simulink model "Flexible_Beam_LP"  (R2014a)
settings: Solver=ode23t  StartTime=0.0  StopTime=200  RelTol=1e-3  AbsTol=1e-6
PreLoadFcn:
  | Cantilever_Beam_MS2G_Parameters
PostLoadFcn:
  | warning off Simulink:Engine:UsingDefaultMaxStepSize
  | warning off Simulink:Engine:SaveWithParameterizedLinks_Warning
undefined symbols (not defined in the file): beam_length, beam_wall, beam_width, Damping, density, Extr_Data_Box, kbendingx, kbendingy, kelongz, ktwistz, num_elem, shearM, X, Y, youngsM, Z
libraries: sm_lib x307, nesl_utility x65
(part 1 of 9)
Description:
  | Copyright 2014 The MathWorks, Inc.
settings Model: Creator=smiller  LastModifiedBy=smiller
settings DebuggingCC: UnderspecifiedInitializationDetection=Classic  StateNameClashWarn=warning
settings ExplorerConfigSet: InternalSimMechanicsExplorerSettings="<ExplorerConfiguration><canonicalview>default</canonicalview><AnimationSetting><BasePlaybackSpeed>1.0</BasePlaybackSpeed><PlaybackSpeedFactor>1.0</PlaybackSpeedFactor></AnimationSetting><TilePanel><TileInfo><Tiles Columns=\"1\" Count=\"1\" Rows=\"1\"><Column Left=\"2\" Weight=\"1\"/><Column Left=\"626\"/><Row Top=\"2\" Weight=\"1\"/><Row Top=\"393\"/><Tile Height=\"1\" Width=\"1\" X=\"0\" Y=\"0\"/></Tiles></TileInfo><SceneInfo><SceneViewer><BGColor><R>0.60000002384185791</R><G>0.60000002384185791</G><B>0.60000002384185791</B></BGColor><Camera><Position><X>46.619711055341185</X><Y>-0.34983005837123721</Y><Z>0.38649668367083467</Z></Position><Center><X>15.061424751729401</X><Y>-0.47805428343950285</Y><Z>0.22325866927449958</Z></Center><Up><X>-0.0040752125209600008</X><Y>0.99998893056788307</Y><Z>0.0023518895830039648</Z></Up><Left>-1.9626362085342408</Left><Right>1.9626362085342408</Right><Bottom>-0.98671855330467229</Bottom><Top>0.98671855330467229</Top></Camera></SceneViewer></SceneInfo></TilePanel></ExplorerConfiguration>"

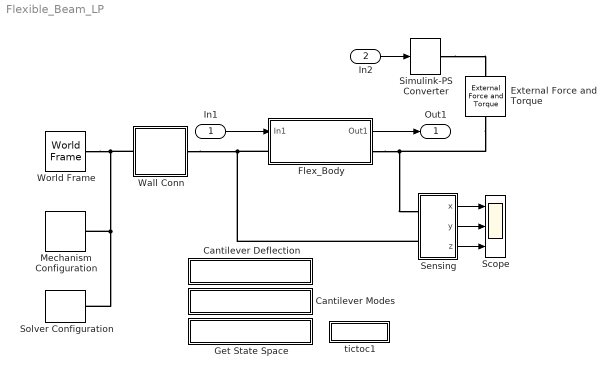
== system Flexible_Beam_LP ==
  In1 : Inport
  In2 : Inport  Port=2
  Cantilever Deflection : Subsystem
      settings: OpenFcn=|
      | mdl = bdroot;
      | 
      | load_system('FlexBeamElement_MS2G_Lib')
      | set_param('FlexBeamElement_MS2G_Lib', 'Lock', 'off');
      | set_param('FlexBeamElement_MS2G_Lib/Flex_Element','BlockChoice','Full')
      | 
      | open_system(mdl);
      | open_system([mdl, '/Scope']);
      | set_param([bdroot '/Wall Conn'],'OverrideUsingVariant','Fixed');
      | %set_param([mdl, '/Sensing/Transform Sensor'],'MeasurementFrame','World')
      | 
      | sim(mdl);
      | disp(['Static Deflection is ' num2str(TipDef.signals(2).values(end)) ' m'])
      mask Display: disp('Cantilever Deflection');
  Cantilever Modes : Subsystem
      settings: OpenFcn=Cantilever_Modes_Shapes_MS2G
      mask Display: disp('Cantilever Modes');
  External Force and Torque : sm_lib/Forces and Torques/External Force and Torque  ForceResolutionFrame=AttachedFrame  EnableForceX=off  EnableForceY=on  EnableForceZ=off  EnableForce=off  TorqueResolutionFrame=AttachedFrame  EnableTorqueX=off  EnableTorqueY=off  EnableTorqueZ=off  EnableTorque=off  BlockFunction=simmechanics.library.forces_torques.external_force_torque
  Flex_Body : Subsystem  mask(Flexible Body){rho=density, youngsM=youngsM, shearM=shearM, numelem=num_elem, beam_length=beam_length, beam_width=beam_width, beam_wall=beam_wall, b=Damping}
      mask prompts: rho "Material Density (kg/(m^3)"; youngsM "Modulus of Elasticity (N/m2)"; shearM "Shear Modulus (N/m2)"; numelem "Number of elements"; beam_length "Beam Length (m)"; beam_width "Beam Width & Height (m)"; beam_wall "Beam Wall Thickness(m)"; b "Damping Constant (Nm/rad.s)"
      mask help:
      | Models a flexible hollow square beam based on lumped parameter method.
      | Number of flexible elements, material properties as well as beam
      | dimension can be varied from mask parameters.
      mask init:
      | [kbendingx, kbendingy, ktwistz, kelongz, length] = Compute_GFE_Prop(rho, youngsM, shearM, numelem, beam_length, beam_width,beam_wall);
      | thisblock = gcb;
      | anno = ['No of Elem: ' num2str(numelem)];
      | set_param(thisblock, 'AttributesFormatString',anno);
      | set_param([thisblock '/Matrix Concatenate'],'NumInputs','numelem')
      | blkchoice = get_param('FlexBeamElement_MS2G_Lib/Flex_Element','BlockChoice');
      | if numelem <1
      |     error('Number of Flexible elements should be greater than 0')
      | end
      | prev_flex_bod = find_system(gcb,'LookUnderMasks','all','RegExp','on','Name','Flex_Elem_*');
      | if ~isempty(prev_flex_bod)
      |     delete_block(prev_flex_bod(1:end))
      | end
      | linehan = find_system(thisblock,'LookUnderMasks','all','FindAll','on','type','line');
      | if ~isempty(linehan)
      |     delete_line(linehan)
      | end
      | blk_or = [100 155 140 195];
      | set_param([thisblock '/B'],'Position',blk_or)
      | set_param([thisblock '/' sprintf('Transform\nBeamX')],'Position',blk_or+[80 0 80 0])
      | add_line(thisblock,['B/Rconn1'],[sprintf('Transform\nBeamX') '/Lconn1'],'autorouting','on');
      | add_block('FlexBeamElement_MS2G_Lib/Flex_Element',[thisblock '/Flex_Elem_' num2str(1)],'Position',blk_or+[80 0 80 0]*2)
      | add_line(thisblock,[sprintf('Transform\nBeamX') '/Rconn1'],['Flex_Elem_' num2str(1) '/Lconn1'],'autorouting','on');
      | add_line(thisblock,'In1/1',['Flex_Elem_' num2str(1) '/1'],'autorouting','on')
      | add_line(thisblock,['Flex_Elem_' num2str(1) '/1'],'Matrix Concatenate/1','autorouting','on')
      | set_param([thisblock '/Flex_Elem_' num2str(1)], 'LinkStatus', 'none')
      | set_param([thisblock '/Flex_Elem_' num2str(1) '/' blkchoice], 'LinkStatus', 'none')
      | set_param([thisblock '/Flex_Elem_' num2str(1) '/' blkchoice '/Selector'],'InputPortWidth','3*numelem')
      | set_param([thisblock '/Flex_Elem_' num2str(1) '/' blkchoice '/Selector'],'Indices','[1 2 3]')
      | if strcmp(blkchoice,'Full')
      |     state_order{1} = [thisblock '/Flex_Elem_' num2str(1) '/' blkchoice '/Bearing Joint'];
      | elseif strcmp(blkchoice,'Elong')
      |     state_order{1} = [thisblock '/Flex_Elem_' num2str(1) '/' blkchoice '/Prismatic Joint'];
      | else
      |     state_order{1} = [thisblock '/Flex_Elem_' num2str(1) '/' blkchoice '/Revolute Joint'];
      | end
      | for i = 2:1:numelem
      |     add_block('FlexBeamElement_MS2G_Lib/Flex_Element',[thisblock '/Flex_Elem_' num2str(i)],'Position',blk_or+(i+1)*[80 0 80 0])
      |     add_line(thisblock,['Flex_Elem_' num2str(i-1) '/Rconn1'],['Flex_Elem_' num2str(i) '/Lconn1'],'autorouting','on');
      |     add_line(thisblock,'In1/1',['Flex_Elem_' num2str(i) '/1'],'autorouting','on')
      |     add_line(thisblock,['Flex_Elem_' num2str(i) '/1'],['Matrix Concatenate/' num2str(i)],'autorouting','on')
      |     set_param([thisblock '/Flex_Elem_' num2str(i)], 'LinkStatus', 'none')
      |     set_param([thisblock '/Flex_Elem_' num2str(i) '/' blkchoice], 'LinkStatus', 'none')
      |     set_param([thisblock '/Flex_Elem_' num2str(i) '/' blkchoice '/Selector'],'InputPortWidth','3*numelem')
      |     set_param([thisblock '/Flex_Elem_' num2str(i) '/' blkchoice '/Selector'],'Indices',['[' num2str([3*i-2 3*i-1 3*i]) ']'])
      |     if strcmp(blkchoice,'Full')
      |         state_order{i} = [thisblock '/Flex_Elem_' num2str(i) '/' blkchoice '/Bearing Joint'];
      |     elseif strcmp(blkchoice,'Elong')
      |         state_order{i} = [thisblock '/Flex_Elem_' num2str(i) '/' blkchoice '/Prismatic Joint'];
      |     else
      |         state_order{i} = [thisblock '/Flex_Elem_' num2str(i) '/' blkchoice '/Revolute Joint'];
      |     end
      | end
      | set_param([thisblock '/F'],'Position',blk_or+ (numelem+2)*[80 0 80 0]);
      | add_line(thisblock,['Flex_Elem_' num2str(numelem) '/Rconn1'],['F/Rconn1'],'autorouting','on');
      | assignin('base','State_order',state_order)
      | add_line(thisblock,'Matrix Concatenate/1','Out1/1','autorouting','on')
      settings: AttributesFormatString=No of Elem: 30  CopyFcn=set_param(gcb, 'LinkStatus', 'none')
      mask Display:
      | image(imread('Flexible_Beam.png'));
      | port_label('input',1,'F_L');
      | port_label('output',1,'wz');
      | color red
      | port_label('LConn',1,'B');
      | port_label('RConn',1,'F');
  Get State Space : Subsystem
      settings: OpenFcn=Cantilever_Linearization_SS_Models
      mask Display: disp('Get State Space');
  Mechanism Configuration : sm_lib/Utilities/Mechanism Configuration  UniformGravity=Constant  GravityVector=gravity  GravityUnits=m/s^2  LinearizationDelta=0.001  BlockFunction=simmechanics.library.utilities.mechanism_configuration
  Scope : Scope  NumInputPorts=3
      settings: YMin=29.8~-1.5~-0.001  YMax=30.2~0~0.001  SaveName=TipDef
  Sensing : Subsystem
  Simulink-PS Converter : nesl_utility/Simulink-PS Converter  PhysicalDomain=network_engine_domain  SubClassName=ps_input  LeftPortType=input  RightPortType=output  PseudoPeriodic=off  Frequencies=[]  NoiseDistribution=none  NoiseParameters=[]  Unit=1  AffineConversion=off  InputFiltering=off  SimscapeFilterOrder=1  InputFilterTimeConstant=0.001  UdotUserProvided=1
  Solver Configuration : nesl_utility/Solver Configuration  PhysicalDomain=network_engine_domain  SubClassName=solver  LeftPortType=input  RightPortType=generic  Accelerate=off  Tones=[]  Harmonics=[]  SimulateNoise=off  Profile=off  UseLocalSampling=off  EnableSwitchedLinearOptims=on  FrequencyDomain=off  UseCCode=off  RelTol=0.001  AbsTol=1e-06  MinStep=1e-09  ToWorkspace=off  DoDC=off  ResidualTolerance=1e-09  UseLocalSolver=off  LocalSolverChoice=NE_BACKWARD_EULER_ADVANCER  LocalSolverSampleTime=0.001  DoFixedCost=off  MaxNonlinIter=3  MaxModeIter=2  LinearAlgebra=Sparse  DelaysMemoryBudget=1024  AutomaticFiltering=on  FilteringTimeConstant=0.001
  Wall Conn : Subsystem  Variant=on  OverrideUsingVariant=Fixed
      mask Display:
      | if strcmp(get_param(gcb,'ActiveVariant'),'Fixed')
      |     image(imread('Weld_Image.png'))
      | else
      |     image(imread('Rev_Image.png'))
      | end
      | color red
      | port_label('LConn',1,'B');
      | port_label('Rconn',1,'F');
  World Frame : sm_lib/Frames and Transforms/World Frame  BlockFunction=simmechanics.library.frames_transforms.world_frame
  tictoc1 : Subsystem
      settings: OpenFcn=open('Flexible_Beam_Demo_Script.html')
      mask Display: disp('Script')
  Out1 : Outport
  wires:
  In2/1 -> Simulink-PS Converter/1
  Sensing/1(x) -> Scope/1
  Sensing/2(y) -> Scope/2
  Sensing/3(z) -> Scope/3
  In1/1 -> Flex_Body/1(In1)
  Flex_Body/1(Out1) -> Out1/1
  connections:
  Simulink-PS Converter/RConn1 -- External Force and Torque/LConn1
  External Force and Torque/RConn1 -- Flex_Body/RConn1 -- Sensing/LConn1
  Solver Configuration/RConn1 -- Wall Conn/LConn1 -- World Frame/RConn1 -- Mechanism Configuration/RConn1
  Sensing/LConn2 -- Flex_Body/LConn1 -- Wall Conn/RConn1

== system Flexible_Beam_LP/Cantilever Deflection ==

== system Flexible_Beam_LP/Cantilever Modes ==

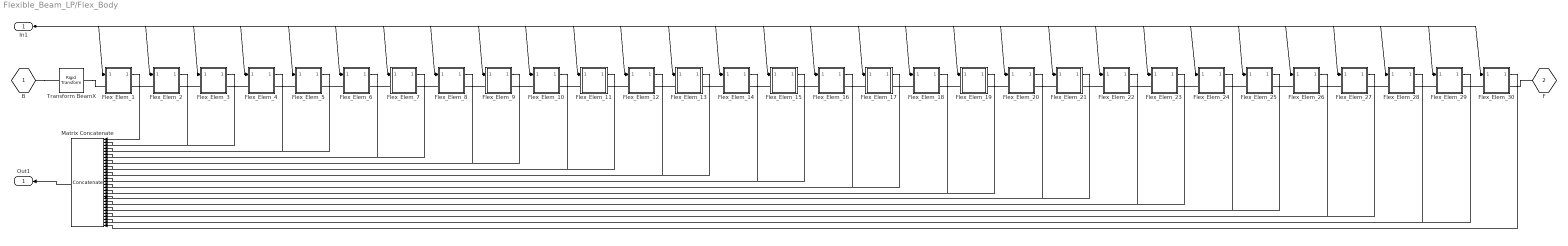
== system Flexible_Beam_LP/Flex_Body ==
  In1 : Inport
  Flex_Elem_1 : Subsystem  BlockChoice=Full
      settings: AttributesFormatString=%<BlockChoice>  TemplateBlock=FlexBeamElement_MS2G_Lib/Flex_Element  MemberBlocks=Bend,Elong,Full
  Flex_Elem_10 : Subsystem  BlockChoice=Full
      settings: AttributesFormatString=%<BlockChoice>  TemplateBlock=FlexBeamElement_MS2G_Lib/Flex_Element  MemberBlocks=Bend,Elong,Full
  Flex_Elem_11 : Subsystem  BlockChoice=Full
      settings: AttributesFormatString=%<BlockChoice>  TemplateBlock=FlexBeamElement_MS2G_Lib/Flex_Element  MemberBlocks=Bend,Elong,Full
  Flex_Elem_12 : Subsystem  BlockChoice=Full
      settings: AttributesFormatString=%<BlockChoice>  TemplateBlock=FlexBeamElement_MS2G_Lib/Flex_Element  MemberBlocks=Bend,Elong,Full
  Flex_Elem_13 : Subsystem  BlockChoice=Full
      settings: AttributesFormatString=%<BlockChoice>  TemplateBlock=FlexBeamElement_MS2G_Lib/Flex_Element  MemberBlocks=Bend,Elong,Full
  Flex_Elem_14 : Subsystem  BlockChoice=Full
      settings: AttributesFormatString=%<BlockChoice>  TemplateBlock=FlexBeamElement_MS2G_Lib/Flex_Element  MemberBlocks=Bend,Elong,Full
  Flex_Elem_15 : Subsystem  BlockChoice=Full
      settings: AttributesFormatString=%<BlockChoice>  TemplateBlock=FlexBeamElement_MS2G_Lib/Flex_Element  MemberBlocks=Bend,Elong,Full
  Flex_Elem_16 : Subsystem  BlockChoice=Full
      settings: AttributesFormatString=%<BlockChoice>  TemplateBlock=FlexBeamElement_MS2G_Lib/Flex_Element  MemberBlocks=Bend,Elong,Full
  Flex_Elem_17 : Subsystem  BlockChoice=Full
      settings: AttributesFormatString=%<BlockChoice>  TemplateBlock=FlexBeamElement_MS2G_Lib/Flex_Element  MemberBlocks=Bend,Elong,Full
  Flex_Elem_18 : Subsystem  BlockChoice=Full
      settings: AttributesFormatString=%<BlockChoice>  TemplateBlock=FlexBeamElement_MS2G_Lib/Flex_Element  MemberBlocks=Bend,Elong,Full
  Flex_Elem_19 : Subsystem  BlockChoice=Full
      settings: AttributesFormatString=%<BlockChoice>  TemplateBlock=FlexBeamElement_MS2G_Lib/Flex_Element  MemberBlocks=Bend,Elong,Full
  Flex_Elem_2 : Subsystem  BlockChoice=Full
      settings: AttributesFormatString=%<BlockChoice>  TemplateBlock=FlexBeamElement_MS2G_Lib/Flex_Element  MemberBlocks=Bend,Elong,Full
  Flex_Elem_20 : Subsystem  BlockChoice=Full
      settings: AttributesFormatString=%<BlockChoice>  TemplateBlock=FlexBeamElement_MS2G_Lib/Flex_Element  MemberBlocks=Bend,Elong,Full
  Flex_Elem_21 : Subsystem  BlockChoice=Full
      settings: AttributesFormatString=%<BlockChoice>  TemplateBlock=FlexBeamElement_MS2G_Lib/Flex_Element  MemberBlocks=Bend,Elong,Full
  Flex_Elem_22 : Subsystem  BlockChoice=Full
      settings: AttributesFormatString=%<BlockChoice>  TemplateBlock=FlexBeamElement_MS2G_Lib/Flex_Element  MemberBlocks=Bend,Elong,Full
  Flex_Elem_23 : Subsystem  BlockChoice=Full
      settings: AttributesFormatString=%<BlockChoice>  TemplateBlock=FlexBeamElement_MS2G_Lib/Flex_Element  MemberBlocks=Bend,Elong,Full
  Flex_Elem_24 : Subsystem  BlockChoice=Full
      settings: AttributesFormatString=%<BlockChoice>  TemplateBlock=FlexBeamElement_MS2G_Lib/Flex_Element  MemberBlocks=Bend,Elong,Full
  Flex_Elem_25 : Subsystem  BlockChoice=Full
      settings: AttributesFormatString=%<BlockChoice>  TemplateBlock=FlexBeamElement_MS2G_Lib/Flex_Element  MemberBlocks=Bend,Elong,Full
  Flex_Elem_26 : Subsystem  BlockChoice=Full
      settings: AttributesFormatString=%<BlockChoice>  TemplateBlock=FlexBeamElement_MS2G_Lib/Flex_Element  MemberBlocks=Bend,Elong,Full
  Flex_Elem_27 : Subsystem  BlockChoice=Full
      settings: AttributesFormatString=%<BlockChoice>  TemplateBlock=FlexBeamElement_MS2G_Lib/Flex_Element  MemberBlocks=Bend,Elong,Full
  Flex_Elem_28 : Subsystem  BlockChoice=Full
      settings: AttributesFormatString=%<BlockChoice>  TemplateBlock=FlexBeamElement_MS2G_Lib/Flex_Element  MemberBlocks=Bend,Elong,Full
  Flex_Elem_29 : Subsystem  BlockChoice=Full
      settings: AttributesFormatString=%<BlockChoice>  TemplateBlock=FlexBeamElement_MS2G_Lib/Flex_Element  MemberBlocks=Bend,Elong,Full
  Flex_Elem_3 : Subsystem  BlockChoice=Full
      settings: AttributesFormatString=%<BlockChoice>  TemplateBlock=FlexBeamElement_MS2G_Lib/Flex_Element  MemberBlocks=Bend,Elong,Full
  Flex_Elem_30 : Subsystem  BlockChoice=Full
      settings: AttributesFormatString=%<BlockChoice>  TemplateBlock=FlexBeamElement_MS2G_Lib/Flex_Element  MemberBlocks=Bend,Elong,Full
  Flex_Elem_4 : Subsystem  BlockChoice=Full
      settings: AttributesFormatString=%<BlockChoice>  TemplateBlock=FlexBeamElement_MS2G_Lib/Flex_Element  MemberBlocks=Bend,Elong,Full
  Flex_Elem_5 : Subsystem  BlockChoice=Full
      settings: AttributesFormatString=%<BlockChoice>  TemplateBlock=FlexBeamElement_MS2G_Lib/Flex_Element  MemberBlocks=Bend,Elong,Full
  Flex_Elem_6 : Subsystem  BlockChoice=Full
      settings: AttributesFormatString=%<BlockChoice>  TemplateBlock=FlexBeamElement_MS2G_Lib/Flex_Element  MemberBlocks=Bend,Elong,Full
  Flex_Elem_7 : Subsystem  BlockChoice=Full
      settings: AttributesFormatString=%<BlockChoice>  TemplateBlock=FlexBeamElement_MS2G_Lib/Flex_Element  MemberBlocks=Bend,Elong,Full
  Flex_Elem_8 : Subsystem  BlockChoice=Full
      settings: AttributesFormatString=%<BlockChoice>  TemplateBlock=FlexBeamElement_MS2G_Lib/Flex_Element  MemberBlocks=Bend,Elong,Full
  Flex_Elem_9 : Subsystem  BlockChoice=Full
      settings: AttributesFormatString=%<BlockChoice>  TemplateBlock=FlexBeamElement_MS2G_Lib/Flex_Element  MemberBlocks=Bend,Elong,Full
  Matrix Concatenate : Concatenate  NumInputs=numelem  Mode=Multidimensional array
  Transform BeamX : sm_lib/Frames and Transforms/Rigid Transform  TranslationMethod=StandardAxis  TranslationLengthUnit=m  TranslationStandardAxis=+Z  TranslationStandardOffset=0  TranslationCartesianOffset=[0 0 0]  TranslationROffset=0  TranslationROffsetUnits=m  TranslationZOffset=0  TranslationZOffsetUnits=m  TranslationThetaOffset=0  TranslationThetaOffsetUnits=deg  RotationMethod=StandardAxis  RotationAngleUnits=deg  RotationStandardAxis=+Y  RotationAngle=90  RotationArbitraryAxis=[0 0 1]  FollAlignAxisA=+X  BaseAlignAxisA=+Y  FollAlignAxisB=+Y  BaseAlignAxisB=+Z  BlockFunction=simmechanics.library.frames_transforms.rigid_transform
  B : PMIOPort  Port=1  Side=Left
  F : PMIOPort  Port=2  Side=Right
  Out1 : Outport
  wires:
  In1/1 -> Flex_Elem_1/1(In1), Flex_Elem_2/1(In1), Flex_Elem_3/1(In1), Flex_Elem_4/1(In1), Flex_Elem_5/1(In1), Flex_Elem_6/1(In1), Flex_Elem_7/1(In1), Flex_Elem_8/1(In1), Flex_Elem_9/1(In1), Flex_Elem_10/1(In1), Flex_Elem_11/1(In1), Flex_Elem_12/1(In1), Flex_Elem_13/1(In1), Flex_Elem_14/1(In1), Flex_Elem_15/1(In1), Flex_Elem_16/1(In1), Flex_Elem_17/1(In1), Flex_Elem_18/1(In1), Flex_Elem_19/1(In1), Flex_Elem_20/1(In1), Flex_Elem_21/1(In1), Flex_Elem_22/1(In1), Flex_Elem_23/1(In1), Flex_Elem_24/1(In1), Flex_Elem_25/1(In1), Flex_Elem_26/1(In1), Flex_Elem_27/1(In1), Flex_Elem_28/1(In1), Flex_Elem_29/1(In1), Flex_Elem_30/1(In1)
  Flex_Elem_1/1(Out1) -> Matrix Concatenate/1
  Flex_Elem_2/1(Out1) -> Matrix Concatenate/2
  Flex_Elem_3/1(Out1) -> Matrix Concatenate/3
  Flex_Elem_4/1(Out1) -> Matrix Concatenate/4
  Flex_Elem_5/1(Out1) -> Matrix Concatenate/5
  Flex_Elem_6/1(Out1) -> Matrix Concatenate/6
  Flex_Elem_7/1(Out1) -> Matrix Concatenate/7
  Flex_Elem_8/1(Out1) -> Matrix Concatenate/8
  Flex_Elem_9/1(Out1) -> Matrix Concatenate/9
  Flex_Elem_10/1(Out1) -> Matrix Concatenate/10
  Flex_Elem_11/1(Out1) -> Matrix Concatenate/11
  Flex_Elem_12/1(Out1) -> Matrix Concatenate/12
  Flex_Elem_13/1(Out1) -> Matrix Concatenate/13
  Flex_Elem_14/1(Out1) -> Matrix Concatenate/14
  Flex_Elem_15/1(Out1) -> Matrix Concatenate/15
  Flex_Elem_16/1(Out1) -> Matrix Concatenate/16
  Flex_Elem_17/1(Out1) -> Matrix Concatenate/17
  Flex_Elem_18/1(Out1) -> Matrix Concatenate/18
  Flex_Elem_19/1(Out1) -> Matrix Concatenate/19
  Flex_Elem_20/1(Out1) -> Matrix Concatenate/20
  Flex_Elem_21/1(Out1) -> Matrix Concatenate/21
  Flex_Elem_22/1(Out1) -> Matrix Concatenate/22
  Flex_Elem_23/1(Out1) -> Matrix Concatenate/23
  Flex_Elem_24/1(Out1) -> Matrix Concatenate/24
  Flex_Elem_25/1(Out1) -> Matrix Concatenate/25
  Flex_Elem_26/1(Out1) -> Matrix Concatenate/26
  Flex_Elem_27/1(Out1) -> Matrix Concatenate/27
  Flex_Elem_28/1(Out1) -> Matrix Concatenate/28
  Flex_Elem_29/1(Out1) -> Matrix Concatenate/29
  Flex_Elem_30/1(Out1) -> Matrix Concatenate/30
  Matrix Concatenate/1 -> Out1/1
  connections:
  B/RConn1 -- Transform BeamX/LConn1
  Transform BeamX/RConn1 -- Flex_Elem_1/LConn1
  Flex_Elem_1/RConn1 -- Flex_Elem_2/LConn1
  Flex_Elem_2/RConn1 -- Flex_Elem_3/LConn1
  Flex_Elem_3/RConn1 -- Flex_Elem_4/LConn1
  Flex_Elem_4/RConn1 -- Flex_Elem_5/LConn1
  Flex_Elem_5/RConn1 -- Flex_Elem_6/LConn1
  Flex_Elem_6/RConn1 -- Flex_Elem_7/LConn1
  Flex_Elem_7/RConn1 -- Flex_Elem_8/LConn1
  Flex_Elem_8/RConn1 -- Flex_Elem_9/LConn1
  Flex_Elem_9/RConn1 -- Flex_Elem_10/LConn1
  Flex_Elem_10/RConn1 -- Flex_Elem_11/LConn1
  Flex_Elem_11/RConn1 -- Flex_Elem_12/LConn1
  Flex_Elem_12/RConn1 -- Flex_Elem_13/LConn1
  Flex_Elem_13/RConn1 -- Flex_Elem_14/LConn1
  Flex_Elem_14/RConn1 -- Flex_Elem_15/LConn1
  Flex_Elem_15/RConn1 -- Flex_Elem_16/LConn1
  Flex_Elem_16/RConn1 -- Flex_Elem_17/LConn1
  Flex_Elem_17/RConn1 -- Flex_Elem_18/LConn1
  Flex_Elem_18/RConn1 -- Flex_Elem_19/LConn1
  Flex_Elem_19/RConn1 -- Flex_Elem_20/LConn1
  Flex_Elem_20/RConn1 -- Flex_Elem_21/LConn1
  Flex_Elem_21/RConn1 -- Flex_Elem_22/LConn1
  Flex_Elem_22/RConn1 -- Flex_Elem_23/LConn1
  Flex_Elem_23/RConn1 -- Flex_Elem_24/LConn1
  Flex_Elem_24/RConn1 -- Flex_Elem_25/LConn1
  Flex_Elem_25/RConn1 -- Flex_Elem_26/LConn1
  Flex_Elem_26/RConn1 -- Flex_Elem_27/LConn1
  Flex_Elem_27/RConn1 -- Flex_Elem_28/LConn1
  Flex_Elem_28/RConn1 -- Flex_Elem_29/LConn1
  Flex_Elem_29/RConn1 -- Flex_Elem_30/LConn1
  Flex_Elem_30/RConn1 -- F/RConn1

== system Flexible_Beam_LP/Get State Space ==

== system Flexible_Beam_LP/Sensing ==
  PS-Simulink Converter : nesl_utility/PS-Simulink Converter  PhysicalDomain=network_engine_domain  SubClassName=ps_output  LeftPortType=input  RightPortType=output  PseudoPeriodic=off  Frequencies=[]  Unit=1  AffineConversion=off
  PS-Simulink Converter1 : nesl_utility/PS-Simulink Converter  PhysicalDomain=network_engine_domain  SubClassName=ps_output  LeftPortType=input  RightPortType=output  PseudoPeriodic=off  Frequencies=[]  Unit=1  AffineConversion=off
  PS-Simulink Converter2 : nesl_utility/PS-Simulink Converter  PhysicalDomain=network_engine_domain  SubClassName=ps_output  LeftPortType=input  RightPortType=output  PseudoPeriodic=off  Frequencies=[]  Unit=1  AffineConversion=off
  Transform Sensor : sm_lib/Frames and Transforms/Transform Sensor  MeasurementFrame=Base  SenseAngle=off  SenseAxis=off  SenseAngle1=off  SenseAngle2=off  SenseAngle3=off  SenseQ=off  SenseR=off  SenseOmegaX=off  SenseOmegaY=off  SenseOmegaZ=off  SenseOmega1=off  SenseOmega2=off  SenseOmega3=off  SenseQDot=off  SenseRDot=off  SenseAlphaX=off  SenseAlphaY=off  SenseAlphaZ=off  SenseAlpha1=off  SenseAlpha2=off  SenseAlpha3=off  SenseQDDot=off  SenseRDDot=off  SenseX=on  SenseY=on  SenseZ=on  SenseRad=off  SenseAzim=off  SenseDist=off  SenseInc=off  SenseXDot=off  SenseYDot=off  SenseZDot=off  SenseRadDot=off  SenseAzimDot=off  SenseDistDot=off  SenseIncDot=off  SenseXDDot=off  SenseYDDot=off  SenseZDDot=off  SenseRadDDot=off  SenseAzimDDot=off  SenseDistDDot=off  SenseIncDDot=off  BlockFunction=simmechanics.library.frames_transforms.transform_sensor
  F : PMIOPort  Port=1  Side=Left
  B : PMIOPort  Port=2  Side=Left
  x : Outport
  y : Outport  Port=2
  z : Outport  Port=3
  wires:
  PS-Simulink Converter1/1 -> y/1
  PS-Simulink Converter2/1 -> z/1
  PS-Simulink Converter/1 -> x/1
  connections:
  PS-Simulink Converter2/LConn1 -- Transform Sensor/RConn4
  PS-Simulink Converter/LConn1 -- Transform Sensor/RConn2
  PS-Simulink Converter1/LConn1 -- Transform Sensor/RConn3
  B/RConn1 -- Transform Sensor/LConn1
  Transform Sensor/RConn1 -- F/RConn1

== system Flexible_Beam_LP/Wall Conn ==
  note: 1) Only subsystems can be added as variant choices at this level
      | 2) Blocks cannot be connected at this level as connectivity is
      | automatically determined at simulation, based on the active variant
  Fixed : Subsystem  VariantControl=Fixed
  Rotate : Subsystem  VariantControl=Rotate
  B : PMIOPort  Port=1  Side=Left
  F : PMIOPort  Port=2  Side=Right

== system Flexible_Beam_LP/tictoc1 ==

== system Flexible_Beam_LP/Flex_Body/Flex_Elem_1 ==
  In1 : Inport
  Full : Subsystem  mask{length=length, rho=rho, beam_width=beam_width, beam_wall=beam_wall, kbendingx=kbendingx, kbendingy=kbendingy, kbendingz=ktwistz, kelongz=kelongz, b=b}
      mask prompts: length "Beam Length (m)"; rho "Material Density (kg/(m^3)"; beam_width "Beam Width & Height (m)"; beam_wall "Beam Wall Thickness (m)"; kbendingx "Bending Spring Constant about X(Nm/rad)"; kbendingy "Bending Spring Constant about Y(Nm/rad)"; kbendingz "Twist Spring Constant about Z(Nm/rad)"; kelongz "Elongation Spring Constant about Z(N/m)"; b "Damping Constant (Nm/rad.s)"
  B : PMIOPort  Port=1  Side=Left
  F : PMIOPort  Port=2  Side=Right
  Out1 : Outport
  wires:
  In1/1 -> Full/1(In1)
  Full/1(Out1) -> Out1/1
  connections:
  Full/LConn1 -- B/RConn1
  Full/RConn1 -- F/RConn1

== system Flexible_Beam_LP/Flex_Body/Flex_Elem_10 ==
  In1 : Inport
  Full : Subsystem  mask{length=length, rho=rho, beam_width=beam_width, beam_wall=beam_wall, kbendingx=kbendingx, kbendingy=kbendingy, kbendingz=ktwistz, kelongz=kelongz, b=b}
      mask prompts: length "Beam Length (m)"; rho "Material Density (kg/(m^3)"; beam_width "Beam Width & Height (m)"; beam_wall "Beam Wall Thickness (m)"; kbendingx "Bending Spring Constant about X(Nm/rad)"; kbendingy "Bending Spring Constant about Y(Nm/rad)"; kbendingz "Twist Spring Constant about Z(Nm/rad)"; kelongz "Elongation Spring Constant about Z(N/m)"; b "Damping Constant (Nm/rad.s)"
  B : PMIOPort  Port=1  Side=Left
  F : PMIOPort  Port=2  Side=Right
  Out1 : Outport
  wires:
  In1/1 -> Full/1(In1)
  Full/1(Out1) -> Out1/1
  connections:
  Full/LConn1 -- B/RConn1
  Full/RConn1 -- F/RConn1

== system Flexible_Beam_LP/Flex_Body/Flex_Elem_11 ==
  In1 : Inport
  Full : Subsystem  mask{length=length, rho=rho, beam_width=beam_width, beam_wall=beam_wall, kbendingx=kbendingx, kbendingy=kbendingy, kbendingz=ktwistz, kelongz=kelongz, b=b}
      mask prompts: length "Beam Length (m)"; rho "Material Density (kg/(m^3)"; beam_width "Beam Width & Height (m)"; beam_wall "Beam Wall Thickness (m)"; kbendingx "Bending Spring Constant about X(Nm/rad)"; kbendingy "Bending Spring Constant about Y(Nm/rad)"; kbendingz "Twist Spring Constant about Z(Nm/rad)"; kelongz "Elongation Spring Constant about Z(N/m)"; b "Damping Constant (Nm/rad.s)"
  B : PMIOPort  Port=1  Side=Left
  F : PMIOPort  Port=2  Side=Right
  Out1 : Outport
  wires:
  In1/1 -> Full/1(In1)
  Full/1(Out1) -> Out1/1
  connections:
  Full/LConn1 -- B/RConn1
  Full/RConn1 -- F/RConn1

== system Flexible_Beam_LP/Flex_Body/Flex_Elem_12 ==
  In1 : Inport
  Full : Subsystem  mask{length=length, rho=rho, beam_width=beam_width, beam_wall=beam_wall, kbendingx=kbendingx, kbendingy=kbendingy, kbendingz=ktwistz, kelongz=kelongz, b=b}
      mask prompts: length "Beam Length (m)"; rho "Material Density (kg/(m^3)"; beam_width "Beam Width & Height (m)"; beam_wall "Beam Wall Thickness (m)"; kbendingx "Bending Spring Constant about X(Nm/rad)"; kbendingy "Bending Spring Constant about Y(Nm/rad)"; kbendingz "Twist Spring Constant about Z(Nm/rad)"; kelongz "Elongation Spring Constant about Z(N/m)"; b "Damping Constant (Nm/rad.s)"
  B : PMIOPort  Port=1  Side=Left
  F : PMIOPort  Port=2  Side=Right
  Out1 : Outport
  wires:
  In1/1 -> Full/1(In1)
  Full/1(Out1) -> Out1/1
  connections:
  Full/LConn1 -- B/RConn1
  Full/RConn1 -- F/RConn1

== system Flexible_Beam_LP/Flex_Body/Flex_Elem_13 ==
  In1 : Inport
  Full : Subsystem  mask{length=length, rho=rho, beam_width=beam_width, beam_wall=beam_wall, kbendingx=kbendingx, kbendingy=kbendingy, kbendingz=ktwistz, kelongz=kelongz, b=b}
      mask prompts: length "Beam Length (m)"; rho "Material Density (kg/(m^3)"; beam_width "Beam Width & Height (m)"; beam_wall "Beam Wall Thickness (m)"; kbendingx "Bending Spring Constant about X(Nm/rad)"; kbendingy "Bending Spring Constant about Y(Nm/rad)"; kbendingz "Twist Spring Constant about Z(Nm/rad)"; kelongz "Elongation Spring Constant about Z(N/m)"; b "Damping Constant (Nm/rad.s)"
  B : PMIOPort  Port=1  Side=Left
  F : PMIOPort  Port=2  Side=Right
  Out1 : Outport
  wires:
  In1/1 -> Full/1(In1)
  Full/1(Out1) -> Out1/1
  connections:
  Full/LConn1 -- B/RConn1
  Full/RConn1 -- F/RConn1

== system Flexible_Beam_LP/Flex_Body/Flex_Elem_14 ==
  In1 : Inport
  Full : Subsystem  mask{length=length, rho=rho, beam_width=beam_width, beam_wall=beam_wall, kbendingx=kbendingx, kbendingy=kbendingy, kbendingz=ktwistz, kelongz=kelongz, b=b}
      mask prompts: length "Beam Length (m)"; rho "Material Density (kg/(m^3)"; beam_width "Beam Width & Height (m)"; beam_wall "Beam Wall Thickness (m)"; kbendingx "Bending Spring Constant about X(Nm/rad)"; kbendingy "Bending Spring Constant about Y(Nm/rad)"; kbendingz "Twist Spring Constant about Z(Nm/rad)"; kelongz "Elongation Spring Constant about Z(N/m)"; b "Damping Constant (Nm/rad.s)"
  B : PMIOPort  Port=1  Side=Left
  F : PMIOPort  Port=2  Side=Right
  Out1 : Outport
  wires:
  In1/1 -> Full/1(In1)
  Full/1(Out1) -> Out1/1
  connections:
  Full/LConn1 -- B/RConn1
  Full/RConn1 -- F/RConn1

== system Flexible_Beam_LP/Flex_Body/Flex_Elem_15 ==
  In1 : Inport
  Full : Subsystem  mask{length=length, rho=rho, beam_width=beam_width, beam_wall=beam_wall, kbendingx=kbendingx, kbendingy=kbendingy, kbendingz=ktwistz, kelongz=kelongz, b=b}
      mask prompts: length "Beam Length (m)"; rho "Material Density (kg/(m^3)"; beam_width "Beam Width & Height (m)"; beam_wall "Beam Wall Thickness (m)"; kbendingx "Bending Spring Constant about X(Nm/rad)"; kbendingy "Bending Spring Constant about Y(Nm/rad)"; kbendingz "Twist Spring Constant about Z(Nm/rad)"; kelongz "Elongation Spring Constant about Z(N/m)"; b "Damping Constant (Nm/rad.s)"
  B : PMIOPort  Port=1  Side=Left
  F : PMIOPort  Port=2  Side=Right
  Out1 : Outport
  wires:
  In1/1 -> Full/1(In1)
  Full/1(Out1) -> Out1/1
  connections:
  Full/LConn1 -- B/RConn1
  Full/RConn1 -- F/RConn1

== system Flexible_Beam_LP/Flex_Body/Flex_Elem_16 ==
  In1 : Inport
  Full : Subsystem  mask{length=length, rho=rho, beam_width=beam_width, beam_wall=beam_wall, kbendingx=kbendingx, kbendingy=kbendingy, kbendingz=ktwistz, kelongz=kelongz, b=b}
      mask prompts: length "Beam Length (m)"; rho "Material Density (kg/(m^3)"; beam_width "Beam Width & Height (m)"; beam_wall "Beam Wall Thickness (m)"; kbendingx "Bending Spring Constant about X(Nm/rad)"; kbendingy "Bending Spring Constant about Y(Nm/rad)"; kbendingz "Twist Spring Constant about Z(Nm/rad)"; kelongz "Elongation Spring Constant about Z(N/m)"; b "Damping Constant (Nm/rad.s)"
  B : PMIOPort  Port=1  Side=Left
  F : PMIOPort  Port=2  Side=Right
  Out1 : Outport
  wires:
  In1/1 -> Full/1(In1)
  Full/1(Out1) -> Out1/1
  connections:
  Full/LConn1 -- B/RConn1
  Full/RConn1 -- F/RConn1

== system Flexible_Beam_LP/Flex_Body/Flex_Elem_17 ==
  In1 : Inport
  Full : Subsystem  mask{length=length, rho=rho, beam_width=beam_width, beam_wall=beam_wall, kbendingx=kbendingx, kbendingy=kbendingy, kbendingz=ktwistz, kelongz=kelongz, b=b}
      mask prompts: length "Beam Length (m)"; rho "Material Density (kg/(m^3)"; beam_width "Beam Width & Height (m)"; beam_wall "Beam Wall Thickness (m)"; kbendingx "Bending Spring Constant about X(Nm/rad)"; kbendingy "Bending Spring Constant about Y(Nm/rad)"; kbendingz "Twist Spring Constant about Z(Nm/rad)"; kelongz "Elongation Spring Constant about Z(N/m)"; b "Damping Constant (Nm/rad.s)"
  B : PMIOPort  Port=1  Side=Left
  F : PMIOPort  Port=2  Side=Right
  Out1 : Outport
  wires:
  In1/1 -> Full/1(In1)
  Full/1(Out1) -> Out1/1
  connections:
  Full/LConn1 -- B/RConn1
  Full/RConn1 -- F/RConn1

== system Flexible_Beam_LP/Flex_Body/Flex_Elem_18 ==
  In1 : Inport
  Full : Subsystem  mask{length=length, rho=rho, beam_width=beam_width, beam_wall=beam_wall, kbendingx=kbendingx, kbendingy=kbendingy, kbendingz=ktwistz, kelongz=kelongz, b=b}
      mask prompts: length "Beam Length (m)"; rho "Material Density (kg/(m^3)"; beam_width "Beam Width & Height (m)"; beam_wall "Beam Wall Thickness (m)"; kbendingx "Bending Spring Constant about X(Nm/rad)"; kbendingy "Bending Spring Constant about Y(Nm/rad)"; kbendingz "Twist Spring Constant about Z(Nm/rad)"; kelongz "Elongation Spring Constant about Z(N/m)"; b "Damping Constant (Nm/rad.s)"
  B : PMIOPort  Port=1  Side=Left
  F : PMIOPort  Port=2  Side=Right
  Out1 : Outport
  wires:
  In1/1 -> Full/1(In1)
  Full/1(Out1) -> Out1/1
  connections:
  Full/LConn1 -- B/RConn1
  Full/RConn1 -- F/RConn1

== system Flexible_Beam_LP/Flex_Body/Flex_Elem_19 ==
  In1 : Inport
  Full : Subsystem  mask{length=length, rho=rho, beam_width=beam_width, beam_wall=beam_wall, kbendingx=kbendingx, kbendingy=kbendingy, kbendingz=ktwistz, kelongz=kelongz, b=b}
      mask prompts: length "Beam Length (m)"; rho "Material Density (kg/(m^3)"; beam_width "Beam Width & Height (m)"; beam_wall "Beam Wall Thickness (m)"; kbendingx "Bending Spring Constant about X(Nm/rad)"; kbendingy "Bending Spring Constant about Y(Nm/rad)"; kbendingz "Twist Spring Constant about Z(Nm/rad)"; kelongz "Elongation Spring Constant about Z(N/m)"; b "Damping Constant (Nm/rad.s)"
  B : PMIOPort  Port=1  Side=Left
  F : PMIOPort  Port=2  Side=Right
  Out1 : Outport
  wires:
  In1/1 -> Full/1(In1)
  Full/1(Out1) -> Out1/1
  connections:
  Full/LConn1 -- B/RConn1
  Full/RConn1 -- F/RConn1

== system Flexible_Beam_LP/Flex_Body/Flex_Elem_2 ==
  In1 : Inport
  Full : Subsystem  mask{length=length, rho=rho, beam_width=beam_width, beam_wall=beam_wall, kbendingx=kbendingx, kbendingy=kbendingy, kbendingz=ktwistz, kelongz=kelongz, b=b}
      mask prompts: length "Beam Length (m)"; rho "Material Density (kg/(m^3)"; beam_width "Beam Width & Height (m)"; beam_wall "Beam Wall Thickness (m)"; kbendingx "Bending Spring Constant about X(Nm/rad)"; kbendingy "Bending Spring Constant about Y(Nm/rad)"; kbendingz "Twist Spring Constant about Z(Nm/rad)"; kelongz "Elongation Spring Constant about Z(N/m)"; b "Damping Constant (Nm/rad.s)"
  B : PMIOPort  Port=1  Side=Left
  F : PMIOPort  Port=2  Side=Right
  Out1 : Outport
  wires:
  In1/1 -> Full/1(In1)
  Full/1(Out1) -> Out1/1
  connections:
  Full/LConn1 -- B/RConn1
  Full/RConn1 -- F/RConn1

== system Flexible_Beam_LP/Flex_Body/Flex_Elem_20 ==
  In1 : Inport
  Full : Subsystem  mask{length=length, rho=rho, beam_width=beam_width, beam_wall=beam_wall, kbendingx=kbendingx, kbendingy=kbendingy, kbendingz=ktwistz, kelongz=kelongz, b=b}
      mask prompts: length "Beam Length (m)"; rho "Material Density (kg/(m^3)"; beam_width "Beam Width & Height (m)"; beam_wall "Beam Wall Thickness (m)"; kbendingx "Bending Spring Constant about X(Nm/rad)"; kbendingy "Bending Spring Constant about Y(Nm/rad)"; kbendingz "Twist Spring Constant about Z(Nm/rad)"; kelongz "Elongation Spring Constant about Z(N/m)"; b "Damping Constant (Nm/rad.s)"
  B : PMIOPort  Port=1  Side=Left
  F : PMIOPort  Port=2  Side=Right
  Out1 : Outport
  wires:
  In1/1 -> Full/1(In1)
  Full/1(Out1) -> Out1/1
  connections:
  Full/LConn1 -- B/RConn1
  Full/RConn1 -- F/RConn1

== system Flexible_Beam_LP/Flex_Body/Flex_Elem_21 ==
  In1 : Inport
  Full : Subsystem  mask{length=length, rho=rho, beam_width=beam_width, beam_wall=beam_wall, kbendingx=kbendingx, kbendingy=kbendingy, kbendingz=ktwistz, kelongz=kelongz, b=b}
      mask prompts: length "Beam Length (m)"; rho "Material Density (kg/(m^3)"; beam_width "Beam Width & Height (m)"; beam_wall "Beam Wall Thickness (m)"; kbendingx "Bending Spring Constant about X(Nm/rad)"; kbendingy "Bending Spring Constant about Y(Nm/rad)"; kbendingz "Twist Spring Constant about Z(Nm/rad)"; kelongz "Elongation Spring Constant about Z(N/m)"; b "Damping Constant (Nm/rad.s)"
  B : PMIOPort  Port=1  Side=Left
  F : PMIOPort  Port=2  Side=Right
  Out1 : Outport
  wires:
  In1/1 -> Full/1(In1)
  Full/1(Out1) -> Out1/1
  connections:
  Full/LConn1 -- B/RConn1
  Full/RConn1 -- F/RConn1

== system Flexible_Beam_LP/Flex_Body/Flex_Elem_22 ==
  In1 : Inport
  Full : Subsystem  mask{length=length, rho=rho, beam_width=beam_width, beam_wall=beam_wall, kbendingx=kbendingx, kbendingy=kbendingy, kbendingz=ktwistz, kelongz=kelongz, b=b}
      mask prompts: length "Beam Length (m)"; rho "Material Density (kg/(m^3)"; beam_width "Beam Width & Height (m)"; beam_wall "Beam Wall Thickness (m)"; kbendingx "Bending Spring Constant about X(Nm/rad)"; kbendingy "Bending Spring Constant about Y(Nm/rad)"; kbendingz "Twist Spring Constant about Z(Nm/rad)"; kelongz "Elongation Spring Constant about Z(N/m)"; b "Damping Constant (Nm/rad.s)"
  B : PMIOPort  Port=1  Side=Left
  F : PMIOPort  Port=2  Side=Right
  Out1 : Outport
  wires:
  In1/1 -> Full/1(In1)
  Full/1(Out1) -> Out1/1
  connections:
  Full/LConn1 -- B/RConn1
  Full/RConn1 -- F/RConn1

== system Flexible_Beam_LP/Flex_Body/Flex_Elem_23 ==
  In1 : Inport
  Full : Subsystem  mask{length=length, rho=rho, beam_width=beam_width, beam_wall=beam_wall, kbendingx=kbendingx, kbendingy=kbendingy, kbendingz=ktwistz, kelongz=kelongz, b=b}
      mask prompts: length "Beam Length (m)"; rho "Material Density (kg/(m^3)"; beam_width "Beam Width & Height (m)"; beam_wall "Beam Wall Thickness (m)"; kbendingx "Bending Spring Constant about X(Nm/rad)"; kbendingy "Bending Spring Constant about Y(Nm/rad)"; kbendingz "Twist Spring Constant about Z(Nm/rad)"; kelongz "Elongation Spring Constant about Z(N/m)"; b "Damping Constant (Nm/rad.s)"
  B : PMIOPort  Port=1  Side=Left
  F : PMIOPort  Port=2  Side=Right
  Out1 : Outport
  wires:
  In1/1 -> Full/1(In1)
  Full/1(Out1) -> Out1/1
  connections:
  Full/LConn1 -- B/RConn1
  Full/RConn1 -- F/RConn1

== system Flexible_Beam_LP/Flex_Body/Flex_Elem_24 ==
  In1 : Inport
  Full : Subsystem  mask{length=length, rho=rho, beam_width=beam_width, beam_wall=beam_wall, kbendingx=kbendingx, kbendingy=kbendingy, kbendingz=ktwistz, kelongz=kelongz, b=b}
      mask prompts: length "Beam Length (m)"; rho "Material Density (kg/(m^3)"; beam_width "Beam Width & Height (m)"; beam_wall "Beam Wall Thickness (m)"; kbendingx "Bending Spring Constant about X(Nm/rad)"; kbendingy "Bending Spring Constant about Y(Nm/rad)"; kbendingz "Twist Spring Constant about Z(Nm/rad)"; kelongz "Elongation Spring Constant about Z(N/m)"; b "Damping Constant (Nm/rad.s)"
  B : PMIOPort  Port=1  Side=Left
  F : PMIOPort  Port=2  Side=Right
  Out1 : Outport
  wires:
  In1/1 -> Full/1(In1)
  Full/1(Out1) -> Out1/1
  connections:
  Full/LConn1 -- B/RConn1
  Full/RConn1 -- F/RConn1

== system Flexible_Beam_LP/Flex_Body/Flex_Elem_25 ==
  In1 : Inport
  Full : Subsystem  mask{length=length, rho=rho, beam_width=beam_width, beam_wall=beam_wall, kbendingx=kbendingx, kbendingy=kbendingy, kbendingz=ktwistz, kelongz=kelongz, b=b}
      mask prompts: length "Beam Length (m)"; rho "Material Density (kg/(m^3)"; beam_width "Beam Width & Height (m)"; beam_wall "Beam Wall Thickness (m)"; kbendingx "Bending Spring Constant about X(Nm/rad)"; kbendingy "Bending Spring Constant about Y(Nm/rad)"; kbendingz "Twist Spring Constant about Z(Nm/rad)"; kelongz "Elongation Spring Constant about Z(N/m)"; b "Damping Constant (Nm/rad.s)"
  B : PMIOPort  Port=1  Side=Left
  F : PMIOPort  Port=2  Side=Right
  Out1 : Outport
  wires:
  In1/1 -> Full/1(In1)
  Full/1(Out1) -> Out1/1
  connections:
  Full/LConn1 -- B/RConn1
  Full/RConn1 -- F/RConn1

== system Flexible_Beam_LP/Flex_Body/Flex_Elem_26 ==
  In1 : Inport
  Full : Subsystem  mask{length=length, rho=rho, beam_width=beam_width, beam_wall=beam_wall, kbendingx=kbendingx, kbendingy=kbendingy, kbendingz=ktwistz, kelongz=kelongz, b=b}
      mask prompts: length "Beam Length (m)"; rho "Material Density (kg/(m^3)"; beam_width "Beam Width & Height (m)"; beam_wall "Beam Wall Thickness (m)"; kbendingx "Bending Spring Constant about X(Nm/rad)"; kbendingy "Bending Spring Constant about Y(Nm/rad)"; kbendingz "Twist Spring Constant about Z(Nm/rad)"; kelongz "Elongation Spring Constant about Z(N/m)"; b "Damping Constant (Nm/rad.s)"
  B : PMIOPort  Port=1  Side=Left
  F : PMIOPort  Port=2  Side=Right
  Out1 : Outport
  wires:
  In1/1 -> Full/1(In1)
  Full/1(Out1) -> Out1/1
  connections:
  Full/LConn1 -- B/RConn1
  Full/RConn1 -- F/RConn1

== system Flexible_Beam_LP/Flex_Body/Flex_Elem_27 ==
  In1 : Inport
  Full : Subsystem  mask{length=length, rho=rho, beam_width=beam_width, beam_wall=beam_wall, kbendingx=kbendingx, kbendingy=kbendingy, kbendingz=ktwistz, kelongz=kelongz, b=b}
      mask prompts: length "Beam Length (m)"; rho "Material Density (kg/(m^3)"; beam_width "Beam Width & Height (m)"; beam_wall "Beam Wall Thickness (m)"; kbendingx "Bending Spring Constant about X(Nm/rad)"; kbendingy "Bending Spring Constant about Y(Nm/rad)"; kbendingz "Twist Spring Constant about Z(Nm/rad)"; kelongz "Elongation Spring Constant about Z(N/m)"; b "Damping Constant (Nm/rad.s)"
  B : PMIOPort  Port=1  Side=Left
  F : PMIOPort  Port=2  Side=Right
  Out1 : Outport
  wires:
  In1/1 -> Full/1(In1)
  Full/1(Out1) -> Out1/1
  connections:
  Full/LConn1 -- B/RConn1
  Full/RConn1 -- F/RConn1

== system Flexible_Beam_LP/Flex_Body/Flex_Elem_28 ==
  In1 : Inport
  Full : Subsystem  mask{length=length, rho=rho, beam_width=beam_width, beam_wall=beam_wall, kbendingx=kbendingx, kbendingy=kbendingy, kbendingz=ktwistz, kelongz=kelongz, b=b}
      mask prompts: length "Beam Length (m)"; rho "Material Density (kg/(m^3)"; beam_width "Beam Width & Height (m)"; beam_wall "Beam Wall Thickness (m)"; kbendingx "Bending Spring Constant about X(Nm/rad)"; kbendingy "Bending Spring Constant about Y(Nm/rad)"; kbendingz "Twist Spring Constant about Z(Nm/rad)"; kelongz "Elongation Spring Constant about Z(N/m)"; b "Damping Constant (Nm/rad.s)"
  B : PMIOPort  Port=1  Side=Left
  F : PMIOPort  Port=2  Side=Right
  Out1 : Outport
  wires:
  In1/1 -> Full/1(In1)
  Full/1(Out1) -> Out1/1
  connections:
  Full/LConn1 -- B/RConn1
  Full/RConn1 -- F/RConn1

== system Flexible_Beam_LP/Flex_Body/Flex_Elem_29 ==
  In1 : Inport
  Full : Subsystem  mask{length=length, rho=rho, beam_width=beam_width, beam_wall=beam_wall, kbendingx=kbendingx, kbendingy=kbendingy, kbendingz=ktwistz, kelongz=kelongz, b=b}
      mask prompts: length "Beam Length (m)"; rho "Material Density (kg/(m^3)"; beam_width "Beam Width & Height (m)"; beam_wall "Beam Wall Thickness (m)"; kbendingx "Bending Spring Constant about X(Nm/rad)"; kbendingy "Bending Spring Constant about Y(Nm/rad)"; kbendingz "Twist Spring Constant about Z(Nm/rad)"; kelongz "Elongation Spring Constant about Z(N/m)"; b "Damping Constant (Nm/rad.s)"
  B : PMIOPort  Port=1  Side=Left
  F : PMIOPort  Port=2  Side=Right
  Out1 : Outport
  wires:
  In1/1 -> Full/1(In1)
  Full/1(Out1) -> Out1/1
  connections:
  Full/LConn1 -- B/RConn1
  Full/RConn1 -- F/RConn1

== system Flexible_Beam_LP/Flex_Body/Flex_Elem_3 ==
  In1 : Inport
  Full : Subsystem  mask{length=length, rho=rho, beam_width=beam_width, beam_wall=beam_wall, kbendingx=kbendingx, kbendingy=kbendingy, kbendingz=ktwistz, kelongz=kelongz, b=b}
      mask prompts: length "Beam Length (m)"; rho "Material Density (kg/(m^3)"; beam_width "Beam Width & Height (m)"; beam_wall "Beam Wall Thickness (m)"; kbendingx "Bending Spring Constant about X(Nm/rad)"; kbendingy "Bending Spring Constant about Y(Nm/rad)"; kbendingz "Twist Spring Constant about Z(Nm/rad)"; kelongz "Elongation Spring Constant about Z(N/m)"; b "Damping Constant (Nm/rad.s)"
  B : PMIOPort  Port=1  Side=Left
  F : PMIOPort  Port=2  Side=Right
  Out1 : Outport
  wires:
  In1/1 -> Full/1(In1)
  Full/1(Out1) -> Out1/1
  connections:
  Full/LConn1 -- B/RConn1
  Full/RConn1 -- F/RConn1

== system Flexible_Beam_LP/Flex_Body/Flex_Elem_30 ==
  In1 : Inport
  Full : Subsystem  mask{length=length, rho=rho, beam_width=beam_width, beam_wall=beam_wall, kbendingx=kbendingx, kbendingy=kbendingy, kbendingz=ktwistz, kelongz=kelongz, b=b}
      mask prompts: length "Beam Length (m)"; rho "Material Density (kg/(m^3)"; beam_width "Beam Width & Height (m)"; beam_wall "Beam Wall Thickness (m)"; kbendingx "Bending Spring Constant about X(Nm/rad)"; kbendingy "Bending Spring Constant about Y(Nm/rad)"; kbendingz "Twist Spring Constant about Z(Nm/rad)"; kelongz "Elongation Spring Constant about Z(N/m)"; b "Damping Constant (Nm/rad.s)"
  B : PMIOPort  Port=1  Side=Left
  F : PMIOPort  Port=2  Side=Right
  Out1 : Outport
  wires:
  In1/1 -> Full/1(In1)
  Full/1(Out1) -> Out1/1
  connections:
  Full/LConn1 -- B/RConn1
  Full/RConn1 -- F/RConn1

== system Flexible_Beam_LP/Flex_Body/Flex_Elem_4 ==
  In1 : Inport
  Full : Subsystem  mask{length=length, rho=rho, beam_width=beam_width, beam_wall=beam_wall, kbendingx=kbendingx, kbendingy=kbendingy, kbendingz=ktwistz, kelongz=kelongz, b=b}
      mask prompts: length "Beam Length (m)"; rho "Material Density (kg/(m^3)"; beam_width "Beam Width & Height (m)"; beam_wall "Beam Wall Thickness (m)"; kbendingx "Bending Spring Constant about X(Nm/rad)"; kbendingy "Bending Spring Constant about Y(Nm/rad)"; kbendingz "Twist Spring Constant about Z(Nm/rad)"; kelongz "Elongation Spring Constant about Z(N/m)"; b "Damping Constant (Nm/rad.s)"
  B : PMIOPort  Port=1  Side=Left
  F : PMIOPort  Port=2  Side=Right
  Out1 : Outport
  wires:
  In1/1 -> Full/1(In1)
  Full/1(Out1) -> Out1/1
  connections:
  Full/LConn1 -- B/RConn1
  Full/RConn1 -- F/RConn1

== system Flexible_Beam_LP/Flex_Body/Flex_Elem_5 ==
  In1 : Inport
  Full : Subsystem  mask{length=length, rho=rho, beam_width=beam_width, beam_wall=beam_wall, kbendingx=kbendingx, kbendingy=kbendingy, kbendingz=ktwistz, kelongz=kelongz, b=b}
      mask prompts: length "Beam Length (m)"; rho "Material Density (kg/(m^3)"; beam_width "Beam Width & Height (m)"; beam_wall "Beam Wall Thickness (m)"; kbendingx "Bending Spring Constant about X(Nm/rad)"; kbendingy "Bending Spring Constant about Y(Nm/rad)"; kbendingz "Twist Spring Constant about Z(Nm/rad)"; kelongz "Elongation Spring Constant about Z(N/m)"; b "Damping Constant (Nm/rad.s)"
  B : PMIOPort  Port=1  Side=Left
  F : PMIOPort  Port=2  Side=Right
  Out1 : Outport
  wires:
  In1/1 -> Full/1(In1)
  Full/1(Out1) -> Out1/1
  connections:
  Full/LConn1 -- B/RConn1
  Full/RConn1 -- F/RConn1

== system Flexible_Beam_LP/Flex_Body/Flex_Elem_6 ==
  In1 : Inport
  Full : Subsystem  mask{length=length, rho=rho, beam_width=beam_width, beam_wall=beam_wall, kbendingx=kbendingx, kbendingy=kbendingy, kbendingz=ktwistz, kelongz=kelongz, b=b}
      mask prompts: length "Beam Length (m)"; rho "Material Density (kg/(m^3)"; beam_width "Beam Width & Height (m)"; beam_wall "Beam Wall Thickness (m)"; kbendingx "Bending Spring Constant about X(Nm/rad)"; kbendingy "Bending Spring Constant about Y(Nm/rad)"; kbendingz "Twist Spring Constant about Z(Nm/rad)"; kelongz "Elongation Spring Constant about Z(N/m)"; b "Damping Constant (Nm/rad.s)"
  B : PMIOPort  Port=1  Side=Left
  F : PMIOPort  Port=2  Side=Right
  Out1 : Outport
  wires:
  In1/1 -> Full/1(In1)
  Full/1(Out1) -> Out1/1
  connections:
  Full/LConn1 -- B/RConn1
  Full/RConn1 -- F/RConn1

== system Flexible_Beam_LP/Flex_Body/Flex_Elem_7 ==
  In1 : Inport
  Full : Subsystem  mask{length=length, rho=rho, beam_width=beam_width, beam_wall=beam_wall, kbendingx=kbendingx, kbendingy=kbendingy, kbendingz=ktwistz, kelongz=kelongz, b=b}
      mask prompts: length "Beam Length (m)"; rho "Material Density (kg/(m^3)"; beam_width "Beam Width & Height (m)"; beam_wall "Beam Wall Thickness (m)"; kbendingx "Bending Spring Constant about X(Nm/rad)"; kbendingy "Bending Spring Constant about Y(Nm/rad)"; kbendingz "Twist Spring Constant about Z(Nm/rad)"; kelongz "Elongation Spring Constant about Z(N/m)"; b "Damping Constant (Nm/rad.s)"
  B : PMIOPort  Port=1  Side=Left
  F : PMIOPort  Port=2  Side=Right
  Out1 : Outport
  wires:
  In1/1 -> Full/1(In1)
  Full/1(Out1) -> Out1/1
  connections:
  Full/LConn1 -- B/RConn1
  Full/RConn1 -- F/RConn1

== system Flexible_Beam_LP/Flex_Body/Flex_Elem_8 ==
  In1 : Inport
  Full : Subsystem  mask{length=length, rho=rho, beam_width=beam_width, beam_wall=beam_wall, kbendingx=kbendingx, kbendingy=kbendingy, kbendingz=ktwistz, kelongz=kelongz, b=b}
      mask prompts: length "Beam Length (m)"; rho "Material Density (kg/(m^3)"; beam_width "Beam Width & Height (m)"; beam_wall "Beam Wall Thickness (m)"; kbendingx "Bending Spring Constant about X(Nm/rad)"; kbendingy "Bending Spring Constant about Y(Nm/rad)"; kbendingz "Twist Spring Constant about Z(Nm/rad)"; kelongz "Elongation Spring Constant about Z(N/m)"; b "Damping Constant (Nm/rad.s)"
  B : PMIOPort  Port=1  Side=Left
  F : PMIOPort  Port=2  Side=Right
  Out1 : Outport
  wires:
  In1/1 -> Full/1(In1)
  Full/1(Out1) -> Out1/1
  connections:
  Full/LConn1 -- B/RConn1
  Full/RConn1 -- F/RConn1

== system Flexible_Beam_LP/Flex_Body/Flex_Elem_9 ==
  In1 : Inport
  Full : Subsystem  mask{length=length, rho=rho, beam_width=beam_width, beam_wall=beam_wall, kbendingx=kbendingx, kbendingy=kbendingy, kbendingz=ktwistz, kelongz=kelongz, b=b}
      mask prompts: length "Beam Length (m)"; rho "Material Density (kg/(m^3)"; beam_width "Beam Width & Height (m)"; beam_wall "Beam Wall Thickness (m)"; kbendingx "Bending Spring Constant about X(Nm/rad)"; kbendingy "Bending Spring Constant about Y(Nm/rad)"; kbendingz "Twist Spring Constant about Z(Nm/rad)"; kelongz "Elongation Spring Constant about Z(N/m)"; b "Damping Constant (Nm/rad.s)"
  B : PMIOPort  Port=1  Side=Left
  F : PMIOPort  Port=2  Side=Right
  Out1 : Outport
  wires:
  In1/1 -> Full/1(In1)
  Full/1(Out1) -> Out1/1
  connections:
  Full/LConn1 -- B/RConn1
  Full/RConn1 -- F/RConn1

== system Flexible_Beam_LP/Wall Conn/Fixed ==
  Weld Joint : sm_lib/Joints/Weld Joint  SenseConstraintForce=off  SenseConstraintForceX=off  SenseConstraintForceY=off  SenseConstraintForceZ=off  SenseConstraintTorque=off  SenseConstraintTorqueX=off  SenseConstraintTorqueY=off  SenseConstraintTorqueZ=off  SenseTotalForce=off  SenseTotalForceX=off  SenseTotalForceY=off  SenseTotalForceZ=off  SenseTotalTorque=off  SenseTotalTorqueX=off  SenseTotalTorqueY=off  SenseTotalTorqueZ=off  CompositeWrenchDir=FollowerOnBase  CompositeWrenchFrame=BaseFrame  BlockFunction=simmechanics.library.joints.weld_joint
  B : PMIOPort  Port=1  Side=Left
  F : PMIOPort  Port=2  Side=Right
  connections:
  F/RConn1 -- Weld Joint/RConn1
  B/RConn1 -- Weld Joint/LConn1
